simulink model "movimientoConDinamica1_2"  (R2014a)
settings: Solver=ode45  StartTime=0.0  StopTime=10.0  RelTol=1e-3
undefined symbols (not defined in the file): sigbuilder_block
libraries: simulink x1
settings Model: Creator=PedroBarquin  LastModifiedBy=PedroBarquin

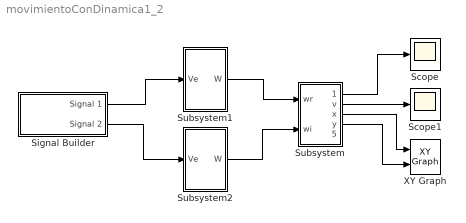
== system movimientoConDinamica1_2 ==
  Scope : Scope
  Scope1 : Scope
  Signal Builder : Subsystem  Tag=STV Subsys  LoadFcn=sigbuilder_block('load',[0.75 23.25 510.75 489 ]);  StartFcn=sigbuilder_block('start');  StopFcn=sigbuilder_block('stop');  ClipboardFcn=sigbuilder_block('clipboard');  mask(Sigbuilder block){}
      mask help: Simulink:masks:SigbuilderBlock_MD
      mask init:
      | if ~strcmp(get_param(bdroot(gcbh),'SimulationStatus'),'stopped') tuvar = sigbuilder_block('maskInit'); end
      settings: CopyFcn=sigbuilder_block('copy');  DeleteFcn=sigbuilder_block('delete');  ModelCloseFcn=sigbuilder_block('modelClose');  PreSaveFcn=sigbuilder_block('preSave');  PauseFcn=sigbuilder_block('pause');  ContinueFcn=sigbuilder_block('continue');  NameChangeFcn=sigbuilder_block('namechange');  OpenFcn=sigbuilder_block('open',[437.6 199.2 550.4 400 ]);  CloseFcn=sigbuilder_block('close');
      mask Display: plot(0, 0, 100, 100,[2, 2, 32, 32, 2], [68, 8, 8, 68, 68],[32, 2], [38, 38], [32, 19, 2],[53, 60, 44], [32, 17, 17, 2],[16, 16, 31, 31]);txt = getActiveGroup(gcbh);text(2, 100, txt,'verticalAlignment', 'top');
  Subsystem : Subsystem  mask{r=1, L=1, x_0=0, y_0=-1, theta_0=0}
  Subsystem1 : Subsystem  mask{A=1, b=1, omega_0=0}
  Subsystem2 : Subsystem  mask{A=1, b=1, omega_0=0}
  XY Graph : simulink/Sinks/XY Graph  xmin=-5  xmax=5  ymin=-5  ymax=5  st=-1
  wires:
  Subsystem/3("x ") -> XY Graph/1
  Subsystem/4("y ") -> XY Graph/2
  Subsystem/2("v ") -> Scope1/1
  Subsystem/1("omega ") -> Scope/1
  Subsystem1/1("W ") -> Subsystem/1("wr ")
  Subsystem2/1("W ") -> Subsystem/2(wi)
  Signal Builder/1(Signal 1) -> Subsystem1/1(Ve)
  Signal Builder/2(Signal 2) -> Subsystem2/1(Ve)

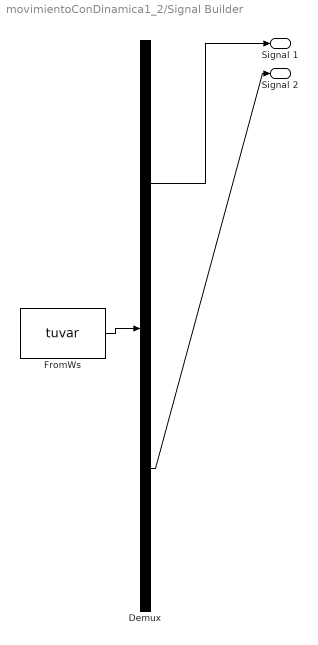
== system movimientoConDinamica1_2/Signal Builder ==
  Demux : Demux  Tag=STV Demux  Outputs=2
  FromWs : FromWorkspace  Tag=STV FromWs  VariableName=tuvar  SampleTime=0
      SigBuilderData=|
      | common.afterFinalStr = 'Extrapolate'
      | common.sampleTime = 0
      | dataSet.timeRange = [0 10]
      | dataSet.name = 'Group 1'
      | sbobj.Groups.Name = 'Group 1'
      | sbobj.Groups.Signals(1).Name = 'Signal 1'
      | sbobj.Groups.Signals(1).XData = [0 1 1 6 10]
      | sbobj.Groups.Signals(1).YData = [0 0 1 1 1]
      | sbobj.Groups.Signals(2).Name = 'Signal 2'
      | sbobj.Groups.Signals(2).XData = [0 1 1 2 2 2.785 2.785 10]
      | sbobj.Groups.Signals(2).YData = [0 0 1 1 -1 -1 1 1]
  Signal 1 : Outport  Tag=STV Outport
  Signal 2 : Outport  Tag=STV Outport  Port=2
  wires:
  Demux/1 -> Signal 1/1
  FromWs/1 -> Demux/1
  Demux/2 -> Signal 2/1

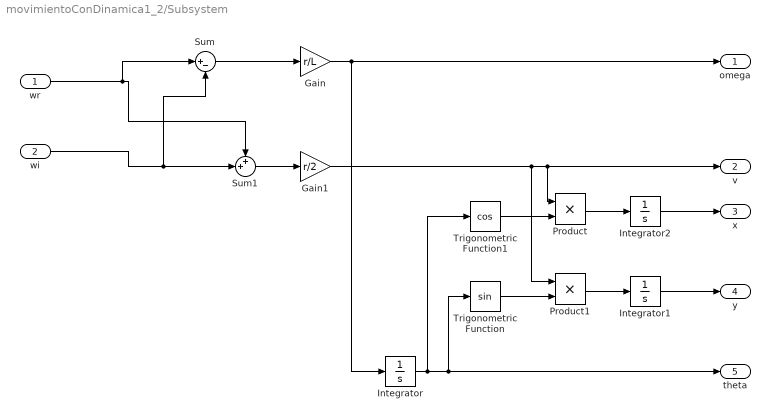
== system movimientoConDinamica1_2/Subsystem ==
  "wr " : Inport
  wi : Inport  Port=2
  Gain : Gain  Gain=r/L
  Gain1 : Gain  Gain=r/2
  Integrator : Integrator  InitialCondition=theta_0
  Integrator1 : Integrator  InitialCondition=y_0
  Integrator2 : Integrator  InitialCondition=x_0
  Product : Product
  Product1 : Product
  Sum : Sum  Inputs=|+-
  Sum1 : Sum  Inputs=++|
  Trigonometric Function : Trigonometry
  Trigonometric Function1 : Trigonometry  Operator=cos
  "omega " : Outport
  "v " : Outport  Port=2
  "x " : Outport  Port=3
  "y " : Outport  Port=4
  "theta " : Outport  Port=5
  wires:
  Gain/1 -> "omega "/1, Integrator/1
  Sum/1 -> Gain/1
  Gain1/1 -> Product1/1, "v "/1, Product/1
  Sum1/1 -> Gain1/1
  wi/1 -> Sum/2, Sum1/2
  "wr "/1 -> Sum/1, Sum1/1
  Trigonometric Function/1 -> Product1/2
  Trigonometric Function1/1 -> Product/2
  Product1/1 -> Integrator1/1
  Integrator/1 -> Trigonometric Function1/1, "theta "/1, Trigonometric Function/1
  Integrator1/1 -> "y "/1
  Product/1 -> Integrator2/1
  Integrator2/1 -> "x "/1

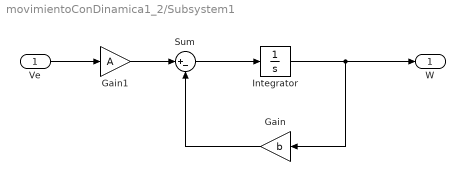
== system movimientoConDinamica1_2/Subsystem1 ==
  Ve : Inport
  Gain : Gain  Gain=b
  Gain1 : Gain  Gain=A
  Integrator : Integrator  InitialCondition=omega_0
  Sum : Sum  Inputs=|+-
  "W " : Outport
  wires:
  Gain1/1 -> Sum/1
  Sum/1 -> Integrator/1
  Ve/1 -> Gain1/1
  Gain/1 -> Sum/2
  Integrator/1 -> "W "/1, Gain/1

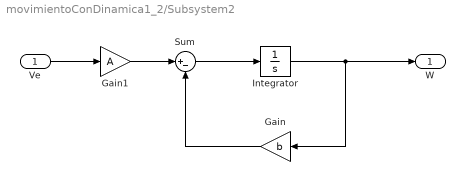
== system movimientoConDinamica1_2/Subsystem2 ==
  Ve : Inport
  Gain : Gain  Gain=b
  Gain1 : Gain  Gain=A
  Integrator : Integrator  InitialCondition=omega_0
  Sum : Sum  Inputs=|+-
  "W " : Outport
  wires:
  Gain1/1 -> Sum/1
  Sum/1 -> Integrator/1
  Ve/1 -> Gain1/1
  Gain/1 -> Sum/2
  Integrator/1 -> "W "/1, Gain/1
